simulink model "New_enth2temp"  (R2013b)
settings: Solver=FixedStepDiscrete  StartTime=0.0  StopTime=10  FixedStep=1  RelTol=1e-3
libraries: carnot x1
settings Model: Creator=awohlfei  LastModifiedBy=awohlfei
settings OptimizationCC: ExpressionDepthLimit=2147483647
settings DebuggingCC: UnderspecifiedInitializationDetection=Simplified  MergeDetectMultiDrivingBlocksExec=error  StateNameClashWarn=warning
settings GRTTargetCC: CombineOutputUpdateFcns=off  GRTInterface=on

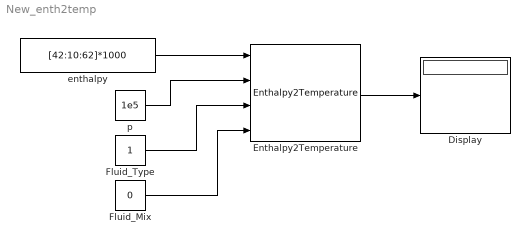
== system New_enth2temp ==
  Display : Display
  Enthalpy2Temperature : carnot/Basic/Material_Properties/Enthalpy2Temperature  VariantControl=CarlibClassic  DEBUGLEVEL=WARNINGLEVEL  MAXTOTALMESSAGES=inf  MAXCONSECUTIVEMESSAGES=inf  WRITETOFILE=0  FILENAME='errors.txt'
  Fluid_Mix : Constant  Value=0
  Fluid_Type : Constant
  enthalpy : Constant  Value=[42:10:62]*1000
  p : Constant  Value=1e5
  wires:
  enthalpy/1 -> Enthalpy2Temperature/1
  Enthalpy2Temperature/1 -> Display/1
  p/1 -> Enthalpy2Temperature/2
  Fluid_Type/1 -> Enthalpy2Temperature/3
  Fluid_Mix/1 -> Enthalpy2Temperature/4
